simulink model "scars_model_lin_test"  (R2019b)
settings: Solver=FixedStepAuto  StartTime=0.0  StopTime=TFinal  FixedStep=dT  RelTol=1e-3
libraries: scars_library x3, simulink x1
settings Model: Creator=asmialek  LastModifiedBy=asmialek

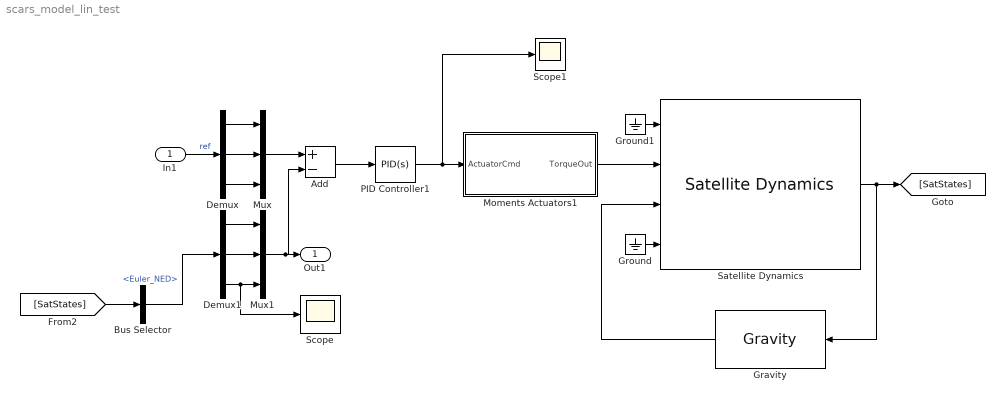
== system scars_model_lin_test ==
  In1 : Inport
  Add : Sum  Inputs=+-
  Bus Selector : BusSelector  OutputSignals=Euler_NED
  Demux : Demux  Outputs=3
  Demux1 : Demux  Outputs=3
  Gravity : scars_library/Environment/Gravity  SystemSampleTime=-1  Latency=0  AutoFrameSizeCalculation=off
  Ground : Ground
  Ground1 : Ground
  Moments Actuators1 : Subsystem
  Mux : Mux  Inputs=3
  Mux1 : Mux  Inputs=3
  PID Controller1 : simulink/Continuous/PID Controller  Controller=PID  Form=Parallel  TimeDomain=Continuous-time  SampleTime=-1  IntegratorMethod=Forward Euler  FilterMethod=Forward Euler  ControllerParametersSource=internal  P=1  I=0  D=5  UseFilter=on  N=100  TunerSelectOption=Transfer Function Based (PID Tuner App)  InitialConditionSource=internal  InitialConditionForIntegrator=0  InitialConditionForFilter=0  DifferentiatorICPrevScaledInput=0  ExternalReset=none  TrackingMode=off  Kt=1  LimitOutput=off  UpperSaturationLimit=inf  LowerSaturationLimit=-inf  LinearizeAsGain=on  AntiWindupMode=none  Kb=1  POutMin=[]  POutMax=[]  IOutMin=[]  IOutMax=[]  DOutMin=[]  DOutMax=[]  NOutMin=[]  NOutMax=[]  SumOutMin=[]  SumOutMax=[]  SaturationOutMin=[]  SaturationOutMax=[]  PParamMin=[]  PParamMax=[]  IParamMin=[]  IParamMax=[]  DParamMin=[]  DParamMax=[]  NParamMin=[]  NParamMax=[]  KbParamMin=[]  KbParamMax=[]  KtParamMin=[]  KtParamMax=[]  KbOutMin=[]  KbOutMax=[]  KtOutMin=[]  KtOutMax=[]  IntegratorOutMin=[]  IntegratorOutMax=[]  FilterOutMin=[]  FilterOutMax=[]  SumI1OutMin=[]  SumI1OutMax=[]  SumI2OutMin=[]  SumI2OutMax=[]  SumI3OutMin=[]  SumI3OutMax=[]  SumI4OutMin=[]  SumI4OutMax=[]  SumDOutMin=[]  SumDOutMax=[]  DifferentiatorOutMin=[]  DifferentiatorOutMax=[]  FilterDiffOutCoefMin=[]  FilterDiffOutCoefMax=[]  ReciprocalOutMin=[]  ReciprocalOutMax=[]  SumDenOutMin=[]  SumDenOutMax=[]  SumNumOutMin=[]  SumNumOutMax=[]  DivideOutMin=[]  DivideOutMax=[]  IntegratorContinuousStateAttributes=''  IntegratorStateMustResolveToSignalObject=off  IntegratorRTWStateStorageClass=Auto  FilterContinuousStateAttributes=''  FilterStateMustResolveToSignalObject=off  FilterRTWStateStorageClass=Auto  ParallelPVariant=InternalParameters  IdealPVariant=Disabled  IVariant=InternalParameters  DVariant=InternalParameters  IntegratorVariant=Continuous  SatVariant=Disabled  AWVariant=Passthrough  PCopyVariant=Disabled  TRVariant=Disabled  FdbkBlocksVariant=Forward  IdealPFdbkVariant=Disabled  SatFdbkVariant=Disabled  DerivativeFilterVariant=ContFilter  NVariant=InternalParameters  NCopyVariant=Disabled  FilterICVariant=InternalICsFilter  IntegratorICVariant=InternalICs  ExternalResetVariant=Disabled  TRSumVariant=Passthrough  SumFdbkVariant=Disabled  SumVariant=Sum_PID
  Satellite Dynamics : scars_library/Advanced/Satellite Dynamics  SystemSampleTime=-1  Latency=0  AutoFrameSizeCalculation=off
      link override Moments Switch/Moments: Value=1
  Scope : Scope
  Scope1 : Scope
  Out1 : Outport
  wires:
  [SatStates] -> Bus Selector/1
  Demux/1 -> Mux/1
  Demux/3 -> Mux/3
  Demux/2 -> Mux/2
  In1/1 -> Demux/1  "ref"
  PID Controller1/1 -> Scope1/1, Moments Actuators1/1(ActuatorCmd)
  Mux/1 -> Add/1
  Add/1 -> PID Controller1/1
  Gravity/1 -> Satellite Dynamics/3
  Ground/1 -> Satellite Dynamics/4
  Ground1/1 -> Satellite Dynamics/1
  Moments Actuators1/1(TorqueOut) -> Satellite Dynamics/2
  Demux1/2 -> Mux1/2
  Demux1/1 -> Mux1/1
  Demux1/3 -> Scope/1, Mux1/3
  Bus Selector/1 -> Demux1/1  "<Euler_NED>"
  Mux1/1 -> Add/2, Out1/1
  Satellite Dynamics/1 -> Gravity/1, [SatStates]

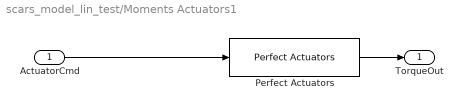
== system scars_model_lin_test/Moments Actuators1 ==
  ActuatorCmd : Inport
  Perfect Actuators : scars_library/Actuators/Perfect Actuators  k=1
  TorqueOut : Outport
  wires:
  Perfect Actuators/1 -> TorqueOut/1
  ActuatorCmd/1 -> Perfect Actuators/1
